simulink model "SimHinfLatdir"  (R2021b)
settings: Solver=VariableStepAuto  StartTime=0.0  StopTime=10.0  RelTol=1e-3
values from neighbouring files (symbols this model uses):
  Alat = modelo.A    [HinfLatDir.m]
  Blat = Blat(:,1)    [HinfLatDir.m]
  Clat = Clat(4,:)    [HinfLatDir.m]
  Dlat = Dlat(4,1)    [HinfLatDir.m]
undefined symbols (not defined in the file or in its folder): K
libraries: simulink x1
settings Model: Creator=Daniel  LastModifiedBy=Daniel

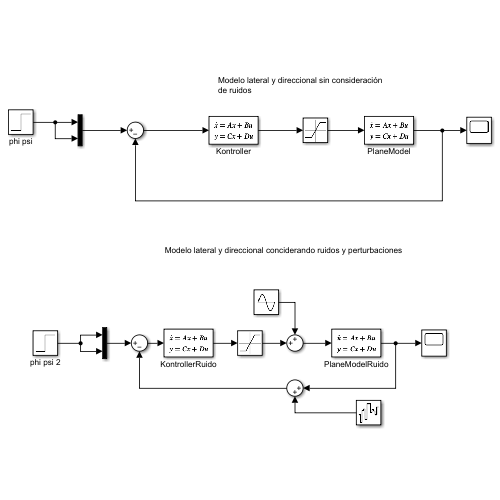
[thumbnail: Simulink's stored preview of the top-level diagram]
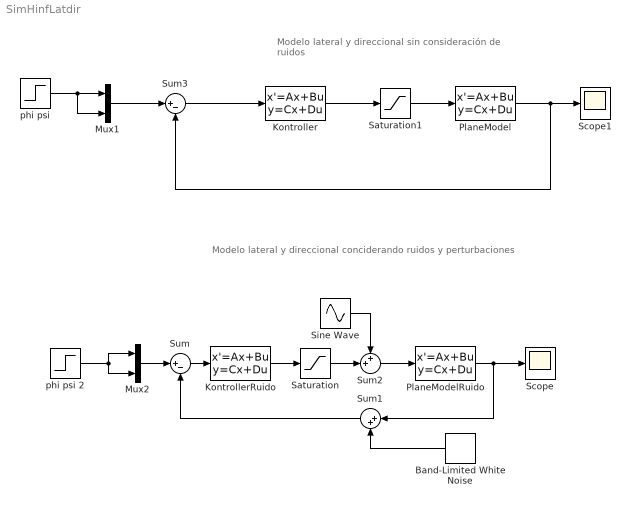
== system SimHinfLatdir ==
  note: Modelo lateral y direccional sin consideración
      | de ruidos
  note: Modelo lateral y direccional conciderando ruidos y perturbaciones
  Band-Limited White Noise : simulink/Sources/Band-Limited White Noise  Cov=[0.0001]  Ts=0.1  seed=[23341]
  Kontroller : StateSpace  A=K.A  B=K.B  C=K.C  D=K.D  InitialCondition=0
  KontrollerRuido : StateSpace  A=K.A  B=K.B  C=K.C  D=K.D  InitialCondition=0
  Mux1 : Mux  Inputs=2
  Mux2 : Mux  Inputs=2
  PlaneModel : StateSpace  A=Alat  B=Blat  C=Clat  D=Dlat  InitialCondition=0
  PlaneModelRuido : StateSpace  A=Alat  B=Blat  C=Clat  D=Dlat  InitialCondition=0
  Saturation : Saturate  UpperLimit=30  LowerLimit=-30
  Saturation1 : Saturate  UpperLimit=30  LowerLimit=-30
  Scope : Scope
  Scope1 : Scope
  Sine Wave : Sin  Frequency=12*pi  SampleTime=0
  Sum : Sum  Inputs=|+-
  Sum1 : Sum  Inputs=|++
  Sum2 : Sum  Inputs=++|
  Sum3 : Sum  Inputs=|+-
  phi psi : Step  Time=0  After=40  SampleTime=0
  phi psi 2 : Step  After=40  SampleTime=0
  wires:
  Sum1/1 -> Sum/2
  Sum/1 -> KontrollerRuido/1
  Saturation/1 -> Sum2/2
  Kontroller/1 -> Saturation1/1
  Sum2/1 -> PlaneModelRuido/1
  PlaneModelRuido/1 -> Sum1/1, Scope/1
  Saturation1/1 -> PlaneModel/1
  Sine Wave/1 -> Sum2/1
  Band-Limited White Noise/1 -> Sum1/2
  KontrollerRuido/1 -> Saturation/1
  PlaneModel/1 -> Sum3/2, Scope1/1
  Sum3/1 -> Kontroller/1
  Mux1/1 -> Sum3/1
  phi psi 2/1 -> Mux2/2, Mux2/1
  Mux2/1 -> Sum/1
  phi psi/1 -> Mux1/2, Mux1/1
